simulink model "backpu"  (R2017b)
settings: Solver=VariableStepAuto  StartTime=0.0  StopTime=10.0  RelTol=1e-3
settings Model: Creator=Truman  LastModifiedBy=Truman

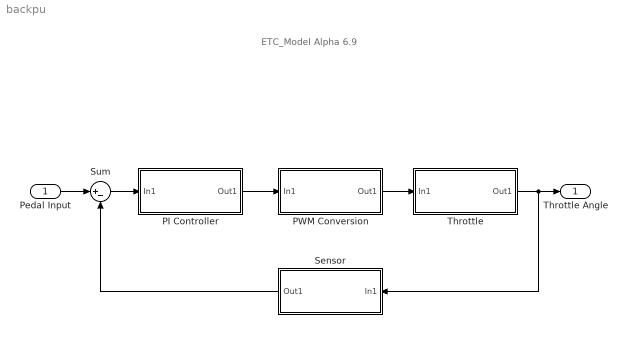
== system backpu ==
  note: ETC_Model Alpha 6.9
  Pedal Input : Inport
  PI Controller : Subsystem  Variant=on
  PWM Conversion : Subsystem  Variant=on
  Sensor : Subsystem  Variant=on
  Sum : Sum  Inputs=|+-
  Throttle : Subsystem  Variant=on
  Throttle Angle : Outport
  wires:
  PI Controller/1(Out1) -> PWM Conversion/1(In1)
  PWM Conversion/1(Out1) -> Throttle/1(In1)
  Throttle/1(Out1) -> Sensor/1(In1), Throttle Angle/1
  Pedal Input/1 -> Sum/1
  Sum/1 -> PI Controller/1(In1)
  Sensor/1(Out1) -> Sum/2

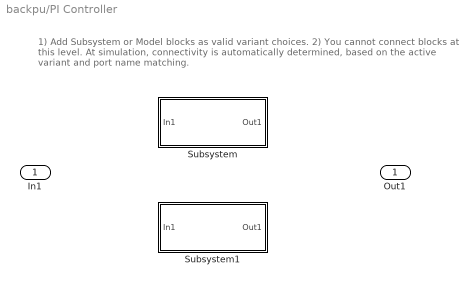
== system backpu/PI Controller ==
  note: 1) Add Subsystem or Model blocks as valid variant choices.
      | 2) You cannot connect blocks at this level. At simulation, connectivity is automatically
      | determined, based on the active variant and port name matching.
  In1 : Inport
  Subsystem : Subsystem  VariantControl=Variant
  Subsystem1 : Subsystem  VariantControl=Variant1
  Out1 : Outport

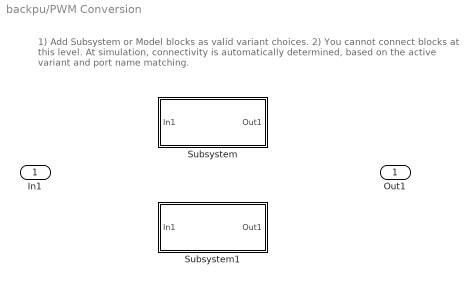
== system backpu/PWM Conversion ==
  note: 1) Add Subsystem or Model blocks as valid variant choices.
      | 2) You cannot connect blocks at this level. At simulation, connectivity is automatically
      | determined, based on the active variant and port name matching.
  In1 : Inport
  Subsystem : Subsystem  VariantControl=Variant
  Subsystem1 : Subsystem  VariantControl=Variant1
  Out1 : Outport

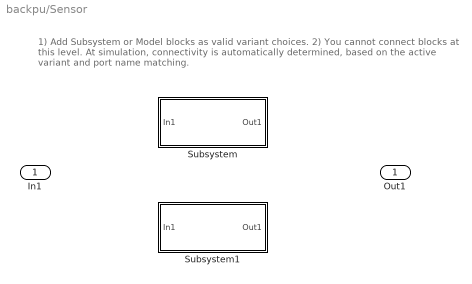
== system backpu/Sensor ==
  note: 1) Add Subsystem or Model blocks as valid variant choices.
      | 2) You cannot connect blocks at this level. At simulation, connectivity is automatically
      | determined, based on the active variant and port name matching.
  In1 : Inport
  Subsystem : Subsystem  VariantControl=Variant
  Subsystem1 : Subsystem  VariantControl=Variant1
  Out1 : Outport

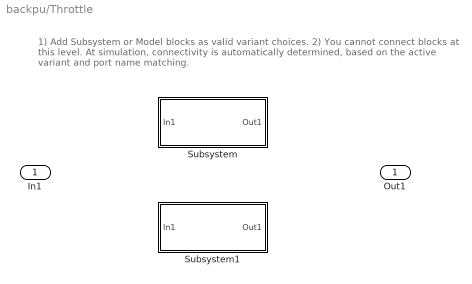
== system backpu/Throttle ==
  note: 1) Add Subsystem or Model blocks as valid variant choices.
      | 2) You cannot connect blocks at this level. At simulation, connectivity is automatically
      | determined, based on the active variant and port name matching.
  In1 : Inport
  Subsystem : Subsystem  VariantControl=Variant
  Subsystem1 : Subsystem  VariantControl=Variant1
  Out1 : Outport

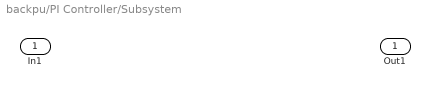
== system backpu/PI Controller/Subsystem ==
  In1 : Inport
  Out1 : Outport

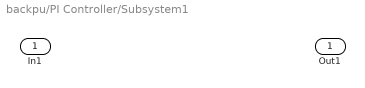
== system backpu/PI Controller/Subsystem1 ==
  In1 : Inport
  Out1 : Outport

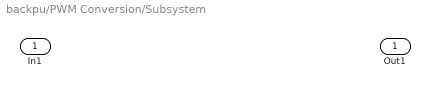
== system backpu/PWM Conversion/Subsystem ==
  In1 : Inport
  Out1 : Outport

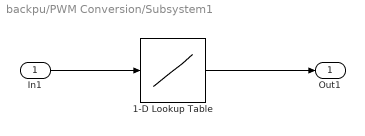
== system backpu/PWM Conversion/Subsystem1 ==
  In1 : Inport
  1-D Lookup Table : Lookup_n-D  NumberOfTableDimensions=1  BreakpointsForDimension1=[-5:5]  Table=tanh([-5:5])  InternalRulePriority=Speed  RndMeth=Simplest  InputSameDT=on
  Out1 : Outport
  wires:
  In1/1 -> 1-D Lookup Table/1
  1-D Lookup Table/1 -> Out1/1

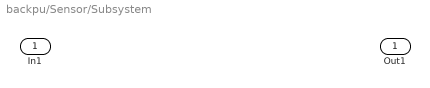
== system backpu/Sensor/Subsystem ==
  In1 : Inport
  Out1 : Outport

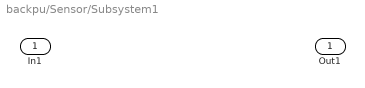
== system backpu/Sensor/Subsystem1 ==
  In1 : Inport
  Out1 : Outport

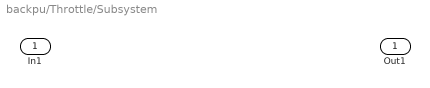
== system backpu/Throttle/Subsystem ==
  In1 : Inport
  Out1 : Outport

== system backpu/Throttle/Subsystem1 ==
  In1 : Inport
  Out1 : Outport
